simulink model "FP_sub_ML2017a"  (R2017a)
settings: Solver=FixedStepAuto  StartTime=0.0  StopTime=T  RelTol=1e-3  EnableMultiTasking=on
values from neighbouring files (symbols this model uses):
  Ts = 1    [Init.m]
libraries: My_FI_Operations x114, simulink x1
settings Model: FPTShortcutValueString='{{},{''BaselineRun'',1,1,1,''BaselineRun'','''',{},''M'',''D'',''''}}'  OrderedModelArguments=off  Creator=kavru  LastModifiedBy=kolbe
settings DataIOCC: ReturnWorkspaceOutputs=on
settings OptimizationCC: BlockReduction=off  ConditionallyExecuteInputs=off
settings DebuggingCC: SignalRangeChecking=warning  SingleTaskRateTransMsg=error
settings SFSimCC: SimUseLocalCustomCode=on
settings RTWCC: RTWUseLocalCustomCode=on

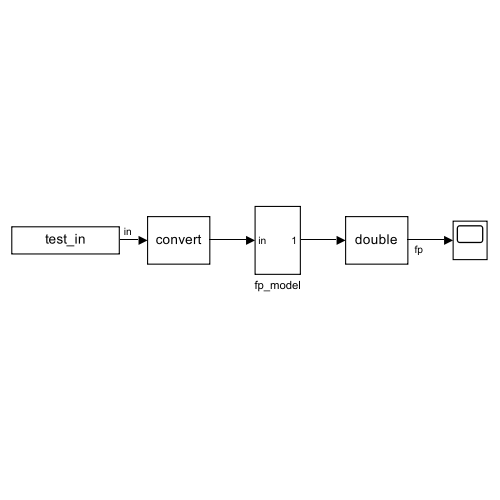
[thumbnail: Simulink's stored preview of the top-level diagram]
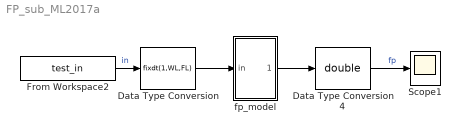
== system FP_sub_ML2017a ==
  Data Type Conversion : DataTypeConversion  OutDataTypeStr=fixdt(1,WL,FL)  RndMeth=Nearest  SaturateOnIntegerOverflow=on
  Data Type Conversion4 : DataTypeConversion  OutDataTypeStr=double  RndMeth=Nearest
  From Workspace2 : FromWorkspace  VariableName=test_in  OutDataTypeStr=double  SampleTime=Ts
  Scope1 : Scope
  fp_model : Subsystem
  wires:
  From Workspace2/1 -> Data Type Conversion/1  "in"
  fp_model/1(Out1) -> Data Type Conversion4/1
  Data Type Conversion/1 -> fp_model/1(in)
  Data Type Conversion4/1 -> Scope1/1  "fp"

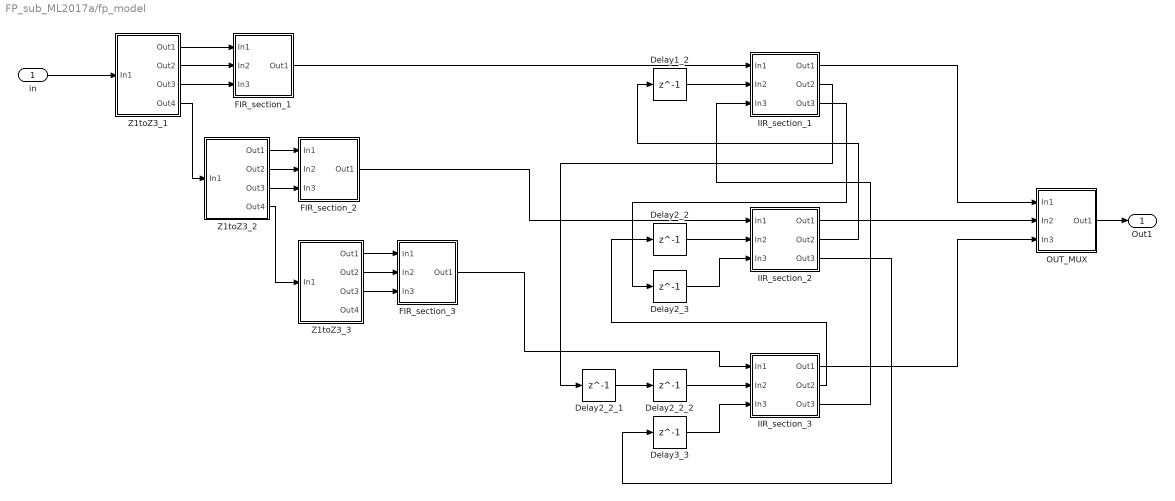
== system FP_sub_ML2017a/fp_model ==
  in : Inport
  Delay1_2 : Delay  DelayLength=1  SampleTime=3*Ts
  Delay2_2 : Delay  DelayLength=1  SampleTime=3*Ts
  Delay2_2_1 : Delay  DelayLength=1  SampleTime=3*Ts
  Delay2_2_2 : Delay  DelayLength=1  SampleTime=3*Ts
  Delay2_3 : Delay  DelayLength=1  SampleTime=3*Ts
  Delay3_3 : Delay  DelayLength=1  SampleTime=3*Ts
  FIR_section_1 : Subsystem
  FIR_section_2 : Subsystem
  FIR_section_3 : Subsystem
  IIR_section_1 : Subsystem
  IIR_section_2 : Subsystem
  IIR_section_3 : Subsystem
  OUT_MUX : Subsystem
  Z1toZ3_1 : Subsystem
  Z1toZ3_2 : Subsystem
  Z1toZ3_3 : Subsystem
  Out1 : Outport
  wires:
  in/1 -> Z1toZ3_1/1(In1)
  Z1toZ3_1/4(Out4) -> Z1toZ3_2/1(In1)
  Z1toZ3_2/4(Out4) -> Z1toZ3_3/1(In1)
  Z1toZ3_1/1(Out1) -> FIR_section_1/1(In1)
  Z1toZ3_1/2(Out2) -> FIR_section_1/2(In2)
  Z1toZ3_1/3(Out3) -> FIR_section_1/3(In3)
  Z1toZ3_2/1(Out1) -> FIR_section_2/1(In1)
  Z1toZ3_2/2(Out2) -> FIR_section_2/2(In2)
  Z1toZ3_2/3(Out3) -> FIR_section_2/3(In3)
  Z1toZ3_3/1(Out1) -> FIR_section_3/1(In1)
  Z1toZ3_3/2(Out2) -> FIR_section_3/2(In2)
  Z1toZ3_3/3(Out3) -> FIR_section_3/3(In3)
  OUT_MUX/1(Out1) -> Out1/1
  FIR_section_1/1(Out1) -> IIR_section_1/1(In1)
  Delay1_2/1 -> IIR_section_1/2(In2)
  IIR_section_1/1(Out1) -> OUT_MUX/1(In1)
  IIR_section_1/3(Out3) -> Delay2_3/1
  FIR_section_2/1(Out1) -> IIR_section_2/1(In1)
  Delay2_3/1 -> IIR_section_2/3(In3)
  Delay2_2/1 -> IIR_section_2/2(In2)
  IIR_section_2/1(Out1) -> OUT_MUX/2(In2)
  IIR_section_2/2(Out2) -> Delay1_2/1
  IIR_section_2/3(Out3) -> Delay3_3/1
  Delay2_2_2/1 -> IIR_section_3/2(In2)
  Delay3_3/1 -> IIR_section_3/3(In3)
  FIR_section_3/1(Out1) -> IIR_section_3/1(In1)
  IIR_section_3/3(Out3) -> IIR_section_1/3(In3)
  IIR_section_3/1(Out1) -> OUT_MUX/3(In3)
  IIR_section_3/2(Out2) -> Delay2_2/1
  Delay2_2_1/1 -> Delay2_2_2/1
  IIR_section_1/2(Out2) -> Delay2_2_1/1

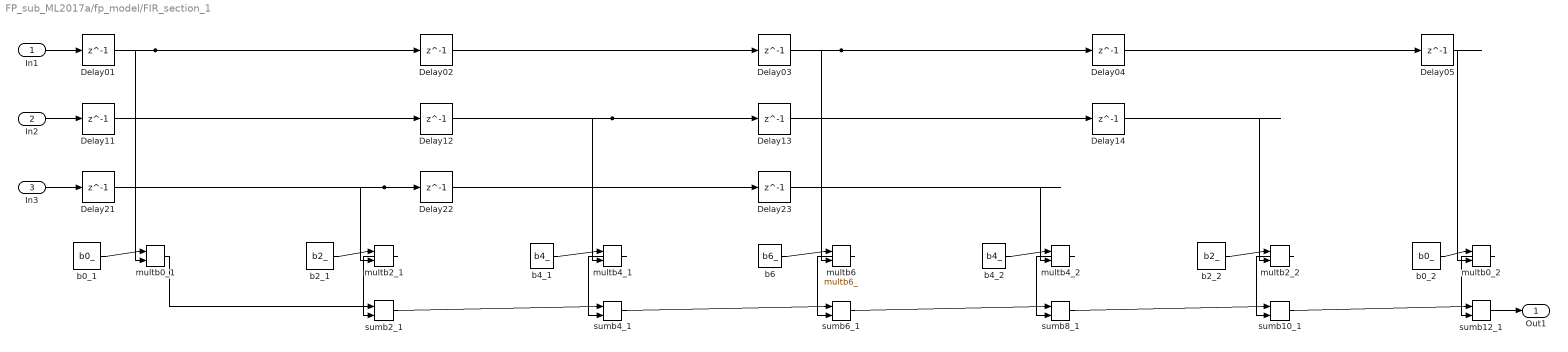
== system FP_sub_ML2017a/fp_model/FIR_section_1 ==
  In1 : Inport
  In2 : Inport  Port=2
  In3 : Inport  Port=3
  Delay01 : Delay  DelayLength=1  SampleTime=3*Ts
  Delay02 : Delay  DelayLength=1  SampleTime=3*Ts
  Delay03 : Delay  DelayLength=1  SampleTime=3*Ts
  Delay04 : Delay  DelayLength=1  SampleTime=3*Ts
  Delay05 : Delay  DelayLength=1  SampleTime=3*Ts
  Delay{11..14,21..23} (7 alike) : Delay  DelayLength=1  SampleTime=3*Ts
  b0_1 : My_FI_Operations/b0_  SystemSampleTime=-1  Latency=0  AutoFrameSizeCalculation=off
  b0_2 : My_FI_Operations/b0_  SystemSampleTime=-1  Latency=0  AutoFrameSizeCalculation=off
  b2_1 : My_FI_Operations/b2_  SystemSampleTime=-1  Latency=0  AutoFrameSizeCalculation=off
  b2_2 : My_FI_Operations/b2_  SystemSampleTime=-1  Latency=0  AutoFrameSizeCalculation=off
  b4_1 : My_FI_Operations/b4_  SystemSampleTime=-1  Latency=0  AutoFrameSizeCalculation=off
  b4_2 : My_FI_Operations/b4_  SystemSampleTime=-1  Latency=0  AutoFrameSizeCalculation=off
  b6 : My_FI_Operations/b6_  SystemSampleTime=-1  Latency=0  AutoFrameSizeCalculation=off
  multb0_1 : My_FI_Operations/multb0_  SystemSampleTime=-1  Latency=0  AutoFrameSizeCalculation=off
  multb0_2 : My_FI_Operations/multb0_  SystemSampleTime=-1  Latency=0  AutoFrameSizeCalculation=off
  multb2_1 : My_FI_Operations/multb2_  SystemSampleTime=-1  Latency=0  AutoFrameSizeCalculation=off
  multb2_2 : My_FI_Operations/multb2_  SystemSampleTime=-1  Latency=0  AutoFrameSizeCalculation=off
  multb4_1 : My_FI_Operations/multb4_  SystemSampleTime=-1  Latency=0  AutoFrameSizeCalculation=off
  multb4_2 : My_FI_Operations/multb4_  SystemSampleTime=-1  Latency=0  AutoFrameSizeCalculation=off
  multb6 : My_FI_Operations/multb6_  SystemSampleTime=-1  Latency=0  AutoFrameSizeCalculation=off
  sumb10_1 : My_FI_Operations/sumb10_  SystemSampleTime=-1  Latency=0  AutoFrameSizeCalculation=off
  sumb12_1 : My_FI_Operations/sumb12_  SystemSampleTime=-1  Latency=0  AutoFrameSizeCalculation=off
  sumb2_1 : My_FI_Operations/sumb2_  SystemSampleTime=-1  Latency=0  AutoFrameSizeCalculation=off
  sumb4_1 : My_FI_Operations/sumb4_  SystemSampleTime=-1  Latency=0  AutoFrameSizeCalculation=off
  sumb6_1 : My_FI_Operations/sumb6_  SystemSampleTime=-1  Latency=0  AutoFrameSizeCalculation=off
  sumb8_1 : My_FI_Operations/sumb8_  SystemSampleTime=-1  Latency=0  AutoFrameSizeCalculation=off
  Out1 : Outport
  wires:
  In3/1 -> Delay21/1
  Delay11/1 -> Delay12/1
  Delay01/1 -> multb0_1/2, Delay02/1
  Delay14/1 -> multb2_2/2
  Delay22/1 -> Delay23/1
  b2_2/1 -> multb2_2/1
  Delay23/1 -> multb4_2/2
  sumb6_1/1 -> sumb8_1/1
  multb2_1/1 -> sumb2_1/2
  Delay13/1 -> Delay14/1
  b0_2/1 -> multb0_2/1
  b0_1/1 -> multb0_1/1
  b4_2/1 -> multb4_2/1
  sumb8_1/1 -> sumb10_1/1
  multb0_2/1 -> sumb12_1/2
  Delay12/1 -> multb4_1/2, Delay13/1
  Delay02/1 -> Delay03/1
  Delay03/1 -> multb6/2, Delay04/1
  sumb4_1/1 -> sumb6_1/1
  multb4_1/1 -> sumb4_1/2
  b6/1 -> multb6/1
  Delay05/1 -> multb0_2/2
  b2_1/1 -> multb2_1/1
  b4_1/1 -> multb4_1/1
  sumb12_1/1 -> Out1/1
  multb6/1 -> sumb6_1/2
  multb0_1/1 -> sumb2_1/1
  multb4_2/1 -> sumb8_1/2
  Delay21/1 -> multb2_1/2, Delay22/1
  sumb2_1/1 -> sumb4_1/1
  In2/1 -> Delay11/1
  multb2_2/1 -> sumb10_1/2
  Delay04/1 -> Delay05/1
  sumb10_1/1 -> sumb12_1/1
  In1/1 -> Delay01/1

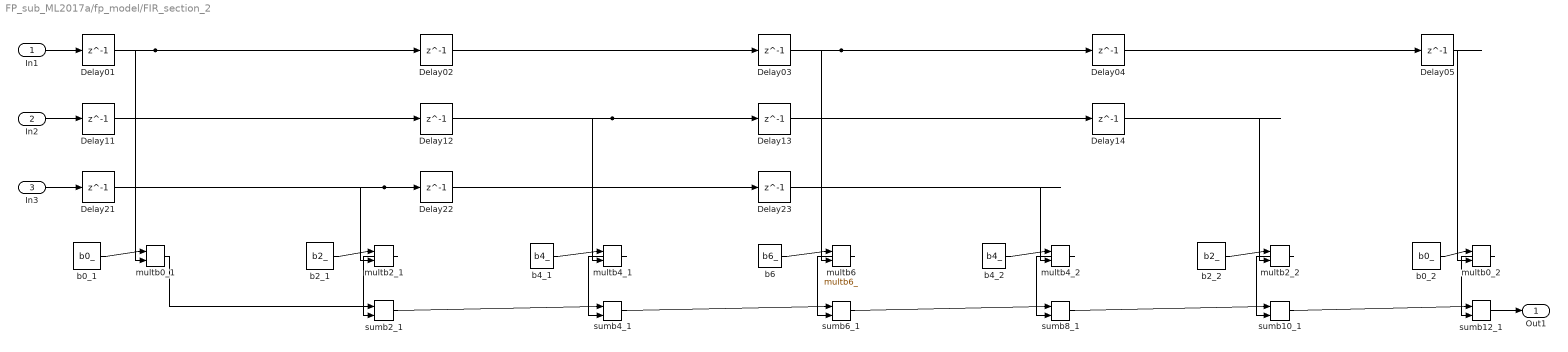
== system FP_sub_ML2017a/fp_model/FIR_section_2 ==
  In1 : Inport
  In2 : Inport  Port=2
  In3 : Inport  Port=3
  Delay01 : Delay  DelayLength=1  SampleTime=3*Ts
  Delay02 : Delay  DelayLength=1  SampleTime=3*Ts
  Delay03 : Delay  DelayLength=1  SampleTime=3*Ts
  Delay04 : Delay  DelayLength=1  SampleTime=3*Ts
  Delay05 : Delay  DelayLength=1  SampleTime=3*Ts
  Delay{11..14,21..23} (7 alike) : Delay  DelayLength=1  SampleTime=3*Ts
  b0_1 : My_FI_Operations/b0_  SystemSampleTime=-1  Latency=0  AutoFrameSizeCalculation=off
  b0_2 : My_FI_Operations/b0_  SystemSampleTime=-1  Latency=0  AutoFrameSizeCalculation=off
  b2_1 : My_FI_Operations/b2_  SystemSampleTime=-1  Latency=0  AutoFrameSizeCalculation=off
  b2_2 : My_FI_Operations/b2_  SystemSampleTime=-1  Latency=0  AutoFrameSizeCalculation=off
  b4_1 : My_FI_Operations/b4_  SystemSampleTime=-1  Latency=0  AutoFrameSizeCalculation=off
  b4_2 : My_FI_Operations/b4_  SystemSampleTime=-1  Latency=0  AutoFrameSizeCalculation=off
  b6 : My_FI_Operations/b6_  SystemSampleTime=-1  Latency=0  AutoFrameSizeCalculation=off
  multb0_1 : My_FI_Operations/multb0_  SystemSampleTime=-1  Latency=0  AutoFrameSizeCalculation=off
  multb0_2 : My_FI_Operations/multb0_  SystemSampleTime=-1  Latency=0  AutoFrameSizeCalculation=off
  multb2_1 : My_FI_Operations/multb2_  SystemSampleTime=-1  Latency=0  AutoFrameSizeCalculation=off
  multb2_2 : My_FI_Operations/multb2_  SystemSampleTime=-1  Latency=0  AutoFrameSizeCalculation=off
  multb4_1 : My_FI_Operations/multb4_  SystemSampleTime=-1  Latency=0  AutoFrameSizeCalculation=off
  multb4_2 : My_FI_Operations/multb4_  SystemSampleTime=-1  Latency=0  AutoFrameSizeCalculation=off
  multb6 : My_FI_Operations/multb6_  SystemSampleTime=-1  Latency=0  AutoFrameSizeCalculation=off
  sumb10_1 : My_FI_Operations/sumb10_  SystemSampleTime=-1  Latency=0  AutoFrameSizeCalculation=off
  sumb12_1 : My_FI_Operations/sumb12_  SystemSampleTime=-1  Latency=0  AutoFrameSizeCalculation=off
  sumb2_1 : My_FI_Operations/sumb2_  SystemSampleTime=-1  Latency=0  AutoFrameSizeCalculation=off
  sumb4_1 : My_FI_Operations/sumb4_  SystemSampleTime=-1  Latency=0  AutoFrameSizeCalculation=off
  sumb6_1 : My_FI_Operations/sumb6_  SystemSampleTime=-1  Latency=0  AutoFrameSizeCalculation=off
  sumb8_1 : My_FI_Operations/sumb8_  SystemSampleTime=-1  Latency=0  AutoFrameSizeCalculation=off
  Out1 : Outport
  wires:
  In3/1 -> Delay21/1
  Delay11/1 -> Delay12/1
  Delay01/1 -> multb0_1/2, Delay02/1
  Delay14/1 -> multb2_2/2
  Delay22/1 -> Delay23/1
  b2_2/1 -> multb2_2/1
  Delay23/1 -> multb4_2/2
  sumb6_1/1 -> sumb8_1/1
  multb2_1/1 -> sumb2_1/2
  Delay13/1 -> Delay14/1
  b0_2/1 -> multb0_2/1
  b0_1/1 -> multb0_1/1
  b4_2/1 -> multb4_2/1
  sumb8_1/1 -> sumb10_1/1
  multb0_2/1 -> sumb12_1/2
  Delay12/1 -> multb4_1/2, Delay13/1
  Delay02/1 -> Delay03/1
  Delay03/1 -> multb6/2, Delay04/1
  sumb4_1/1 -> sumb6_1/1
  multb4_1/1 -> sumb4_1/2
  b6/1 -> multb6/1
  Delay05/1 -> multb0_2/2
  b2_1/1 -> multb2_1/1
  b4_1/1 -> multb4_1/1
  sumb12_1/1 -> Out1/1
  multb6/1 -> sumb6_1/2
  multb0_1/1 -> sumb2_1/1
  multb4_2/1 -> sumb8_1/2
  Delay21/1 -> multb2_1/2, Delay22/1
  sumb2_1/1 -> sumb4_1/1
  In2/1 -> Delay11/1
  multb2_2/1 -> sumb10_1/2
  Delay04/1 -> Delay05/1
  sumb10_1/1 -> sumb12_1/1
  In1/1 -> Delay01/1

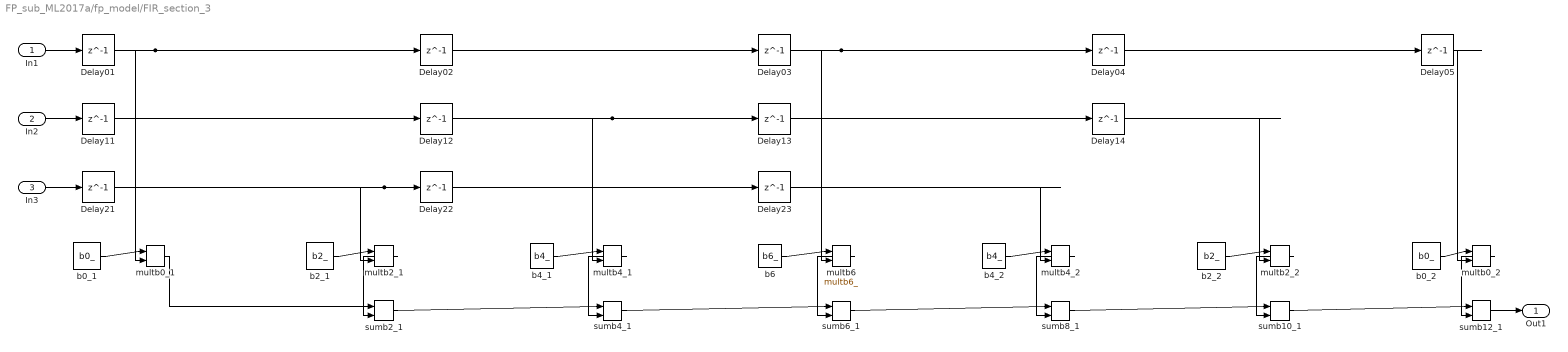
== system FP_sub_ML2017a/fp_model/FIR_section_3 ==
  In1 : Inport
  In2 : Inport  Port=2
  In3 : Inport  Port=3
  Delay01 : Delay  DelayLength=1  SampleTime=3*Ts
  Delay02 : Delay  DelayLength=1  SampleTime=3*Ts
  Delay03 : Delay  DelayLength=1  SampleTime=3*Ts
  Delay04 : Delay  DelayLength=1  SampleTime=3*Ts
  Delay05 : Delay  DelayLength=1  SampleTime=3*Ts
  Delay{11..14,21..23} (7 alike) : Delay  DelayLength=1  SampleTime=3*Ts
  b0_1 : My_FI_Operations/b0_  SystemSampleTime=-1  Latency=0  AutoFrameSizeCalculation=off
  b0_2 : My_FI_Operations/b0_  SystemSampleTime=-1  Latency=0  AutoFrameSizeCalculation=off
  b2_1 : My_FI_Operations/b2_  SystemSampleTime=-1  Latency=0  AutoFrameSizeCalculation=off
  b2_2 : My_FI_Operations/b2_  SystemSampleTime=-1  Latency=0  AutoFrameSizeCalculation=off
  b4_1 : My_FI_Operations/b4_  SystemSampleTime=-1  Latency=0  AutoFrameSizeCalculation=off
  b4_2 : My_FI_Operations/b4_  SystemSampleTime=-1  Latency=0  AutoFrameSizeCalculation=off
  b6 : My_FI_Operations/b6_  SystemSampleTime=-1  Latency=0  AutoFrameSizeCalculation=off
  multb0_1 : My_FI_Operations/multb0_  SystemSampleTime=-1  Latency=0  AutoFrameSizeCalculation=off
  multb0_2 : My_FI_Operations/multb0_  SystemSampleTime=-1  Latency=0  AutoFrameSizeCalculation=off
  multb2_1 : My_FI_Operations/multb2_  SystemSampleTime=-1  Latency=0  AutoFrameSizeCalculation=off
  multb2_2 : My_FI_Operations/multb2_  SystemSampleTime=-1  Latency=0  AutoFrameSizeCalculation=off
  multb4_1 : My_FI_Operations/multb4_  SystemSampleTime=-1  Latency=0  AutoFrameSizeCalculation=off
  multb4_2 : My_FI_Operations/multb4_  SystemSampleTime=-1  Latency=0  AutoFrameSizeCalculation=off
  multb6 : My_FI_Operations/multb6_  SystemSampleTime=-1  Latency=0  AutoFrameSizeCalculation=off
  sumb10_1 : My_FI_Operations/sumb10_  SystemSampleTime=-1  Latency=0  AutoFrameSizeCalculation=off
  sumb12_1 : My_FI_Operations/sumb12_  SystemSampleTime=-1  Latency=0  AutoFrameSizeCalculation=off
  sumb2_1 : My_FI_Operations/sumb2_  SystemSampleTime=-1  Latency=0  AutoFrameSizeCalculation=off
  sumb4_1 : My_FI_Operations/sumb4_  SystemSampleTime=-1  Latency=0  AutoFrameSizeCalculation=off
  sumb6_1 : My_FI_Operations/sumb6_  SystemSampleTime=-1  Latency=0  AutoFrameSizeCalculation=off
  sumb8_1 : My_FI_Operations/sumb8_  SystemSampleTime=-1  Latency=0  AutoFrameSizeCalculation=off
  Out1 : Outport
  wires:
  In3/1 -> Delay21/1
  Delay11/1 -> Delay12/1
  Delay01/1 -> multb0_1/2, Delay02/1
  Delay14/1 -> multb2_2/2
  Delay22/1 -> Delay23/1
  b2_2/1 -> multb2_2/1
  Delay23/1 -> multb4_2/2
  sumb6_1/1 -> sumb8_1/1
  multb2_1/1 -> sumb2_1/2
  Delay13/1 -> Delay14/1
  b0_2/1 -> multb0_2/1
  b0_1/1 -> multb0_1/1
  b4_2/1 -> multb4_2/1
  sumb8_1/1 -> sumb10_1/1
  multb0_2/1 -> sumb12_1/2
  Delay12/1 -> multb4_1/2, Delay13/1
  Delay02/1 -> Delay03/1
  Delay03/1 -> multb6/2, Delay04/1
  sumb4_1/1 -> sumb6_1/1
  multb4_1/1 -> sumb4_1/2
  b6/1 -> multb6/1
  Delay05/1 -> multb0_2/2
  b2_1/1 -> multb2_1/1
  b4_1/1 -> multb4_1/1
  sumb12_1/1 -> Out1/1
  multb6/1 -> sumb6_1/2
  multb0_1/1 -> sumb2_1/1
  multb4_2/1 -> sumb8_1/2
  Delay21/1 -> multb2_1/2, Delay22/1
  sumb2_1/1 -> sumb4_1/1
  In2/1 -> Delay11/1
  multb2_2/1 -> sumb10_1/2
  Delay04/1 -> Delay05/1
  sumb10_1/1 -> sumb12_1/1
  In1/1 -> Delay01/1

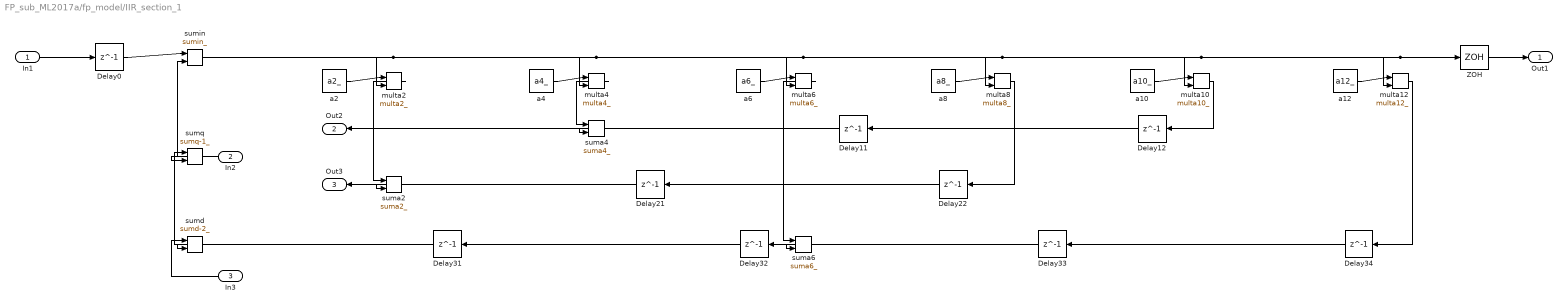
== system FP_sub_ML2017a/fp_model/IIR_section_1 ==
  In1 : Inport
  In2 : Inport  Port=2
  In3 : Inport  Port=3
  Delay{0,11..12,21..22,31..34} (9 alike) : Delay  DelayLength=1  SampleTime=3*Ts
  ZOH : ZeroOrderHold  SampleTime=3*Ts
  a10 : My_FI_Operations/a10_  SystemSampleTime=-1  Latency=0  AutoFrameSizeCalculation=off
  a12 : My_FI_Operations/a12_  SystemSampleTime=-1  Latency=0  AutoFrameSizeCalculation=off
  a2 : My_FI_Operations/a2_  SystemSampleTime=-1  Latency=0  AutoFrameSizeCalculation=off
  a4 : My_FI_Operations/a4_  SystemSampleTime=-1  Latency=0  AutoFrameSizeCalculation=off
  a6 : My_FI_Operations/a6_  SystemSampleTime=-1  Latency=0  AutoFrameSizeCalculation=off
  a8 : My_FI_Operations/a8_  SystemSampleTime=-1  Latency=0  AutoFrameSizeCalculation=off
  multa10 : My_FI_Operations/multa10_  SystemSampleTime=-1  Latency=0  AutoFrameSizeCalculation=off
  multa12 : My_FI_Operations/multa12_  SystemSampleTime=-1  Latency=0  AutoFrameSizeCalculation=off
  multa2 : My_FI_Operations/multa2_  SystemSampleTime=-1  Latency=0  AutoFrameSizeCalculation=off
  multa4 : My_FI_Operations/multa4_  SystemSampleTime=-1  Latency=0  AutoFrameSizeCalculation=off
  multa6 : My_FI_Operations/multa6_  SystemSampleTime=-1  Latency=0  AutoFrameSizeCalculation=off
  multa8 : My_FI_Operations/multa8_  SystemSampleTime=-1  Latency=0  AutoFrameSizeCalculation=off
  suma2 : My_FI_Operations/suma2_  SystemSampleTime=-1  Latency=0  AutoFrameSizeCalculation=off
  suma4 : My_FI_Operations/suma4_  SystemSampleTime=-1  Latency=0  AutoFrameSizeCalculation=off
  suma6 : My_FI_Operations/suma6_  SystemSampleTime=-1  Latency=0  AutoFrameSizeCalculation=off
  sumd : My_FI_Operations/sumd-2_  SystemSampleTime=-1  Latency=0  AutoFrameSizeCalculation=off
  sumin : My_FI_Operations/sumin_  SystemSampleTime=-1  Latency=0  AutoFrameSizeCalculation=off
  sumq : My_FI_Operations/sumq-1_  SystemSampleTime=-1  Latency=0  AutoFrameSizeCalculation=off
  Out1 : Outport
  Out2 : Outport  Port=2
  Out3 : Outport  Port=3
  wires:
  Delay0/1 -> sumin/1
  a12/1 -> multa12/1
  Delay22/1 -> Delay21/1
  Delay31/1 -> sumd/2
  sumin/1 -> multa2/2, multa4/2, multa6/2, multa8/2, multa10/2, multa12/2, ZOH/1
  Delay33/1 -> suma6/2
  Delay32/1 -> Delay31/1
  Delay21/1 -> suma2/2
  sumd/1 -> sumq/1
  a2/1 -> multa2/1
  multa4/1 -> suma4/1
  Delay12/1 -> Delay11/1
  ZOH/1 -> Out1/1
  multa6/1 -> suma6/1
  a10/1 -> multa10/1
  a4/1 -> multa4/1
  multa12/1 -> Delay34/1
  multa2/1 -> suma2/1
  Delay34/1 -> Delay33/1
  a8/1 -> multa8/1
  suma6/1 -> Delay32/1
  Delay11/1 -> suma4/2
  multa10/1 -> Delay12/1
  multa8/1 -> Delay22/1
  sumq/1 -> sumin/2
  a6/1 -> multa6/1
  In2/1 -> sumq/2
  In1/1 -> Delay0/1
  In3/1 -> sumd/1
  suma2/1 -> Out3/1
  suma4/1 -> Out2/1

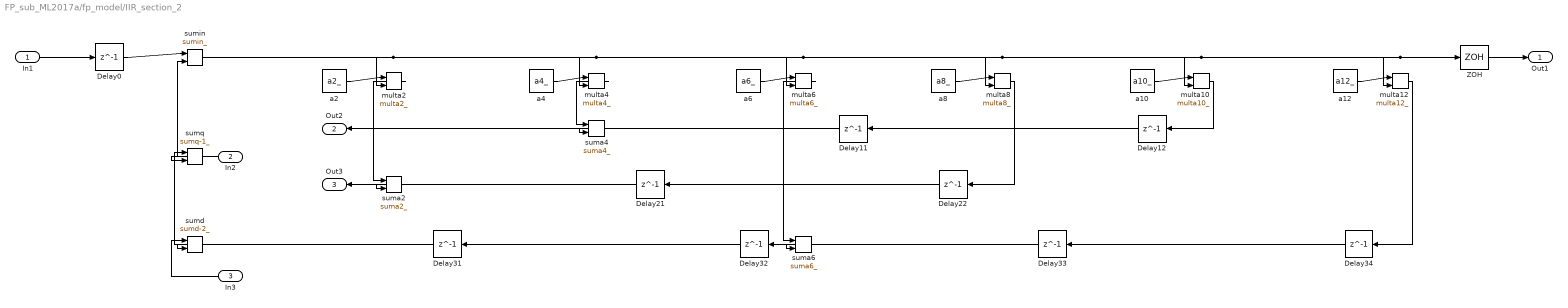
== system FP_sub_ML2017a/fp_model/IIR_section_2 ==
  In1 : Inport
  In2 : Inport  Port=2
  In3 : Inport  Port=3
  Delay{0,11..12,21..22,31..34} (9 alike) : Delay  DelayLength=1  SampleTime=3*Ts
  ZOH : ZeroOrderHold  SampleTime=3*Ts
  a10 : My_FI_Operations/a10_  SystemSampleTime=-1  Latency=0  AutoFrameSizeCalculation=off
  a12 : My_FI_Operations/a12_  SystemSampleTime=-1  Latency=0  AutoFrameSizeCalculation=off
  a2 : My_FI_Operations/a2_  SystemSampleTime=-1  Latency=0  AutoFrameSizeCalculation=off
  a4 : My_FI_Operations/a4_  SystemSampleTime=-1  Latency=0  AutoFrameSizeCalculation=off
  a6 : My_FI_Operations/a6_  SystemSampleTime=-1  Latency=0  AutoFrameSizeCalculation=off
  a8 : My_FI_Operations/a8_  SystemSampleTime=-1  Latency=0  AutoFrameSizeCalculation=off
  multa10 : My_FI_Operations/multa10_  SystemSampleTime=-1  Latency=0  AutoFrameSizeCalculation=off
  multa12 : My_FI_Operations/multa12_  SystemSampleTime=-1  Latency=0  AutoFrameSizeCalculation=off
  multa2 : My_FI_Operations/multa2_  SystemSampleTime=-1  Latency=0  AutoFrameSizeCalculation=off
  multa4 : My_FI_Operations/multa4_  SystemSampleTime=-1  Latency=0  AutoFrameSizeCalculation=off
  multa6 : My_FI_Operations/multa6_  SystemSampleTime=-1  Latency=0  AutoFrameSizeCalculation=off
  multa8 : My_FI_Operations/multa8_  SystemSampleTime=-1  Latency=0  AutoFrameSizeCalculation=off
  suma2 : My_FI_Operations/suma2_  SystemSampleTime=-1  Latency=0  AutoFrameSizeCalculation=off
  suma4 : My_FI_Operations/suma4_  SystemSampleTime=-1  Latency=0  AutoFrameSizeCalculation=off
  suma6 : My_FI_Operations/suma6_  SystemSampleTime=-1  Latency=0  AutoFrameSizeCalculation=off
  sumd : My_FI_Operations/sumd-2_  SystemSampleTime=-1  Latency=0  AutoFrameSizeCalculation=off
  sumin : My_FI_Operations/sumin_  SystemSampleTime=-1  Latency=0  AutoFrameSizeCalculation=off
  sumq : My_FI_Operations/sumq-1_  SystemSampleTime=-1  Latency=0  AutoFrameSizeCalculation=off
  Out1 : Outport
  Out2 : Outport  Port=2
  Out3 : Outport  Port=3
  wires:
  Delay0/1 -> sumin/1
  a12/1 -> multa12/1
  Delay22/1 -> Delay21/1
  Delay31/1 -> sumd/2
  sumin/1 -> multa2/2, multa4/2, multa6/2, multa8/2, multa10/2, multa12/2, ZOH/1
  Delay33/1 -> suma6/2
  Delay32/1 -> Delay31/1
  Delay21/1 -> suma2/2
  sumd/1 -> sumq/1
  a2/1 -> multa2/1
  multa4/1 -> suma4/1
  Delay12/1 -> Delay11/1
  ZOH/1 -> Out1/1
  multa6/1 -> suma6/1
  a10/1 -> multa10/1
  a4/1 -> multa4/1
  multa12/1 -> Delay34/1
  multa2/1 -> suma2/1
  Delay34/1 -> Delay33/1
  a8/1 -> multa8/1
  suma6/1 -> Delay32/1
  Delay11/1 -> suma4/2
  multa10/1 -> Delay12/1
  multa8/1 -> Delay22/1
  sumq/1 -> sumin/2
  a6/1 -> multa6/1
  In2/1 -> sumq/2
  In1/1 -> Delay0/1
  In3/1 -> sumd/1
  suma2/1 -> Out3/1
  suma4/1 -> Out2/1

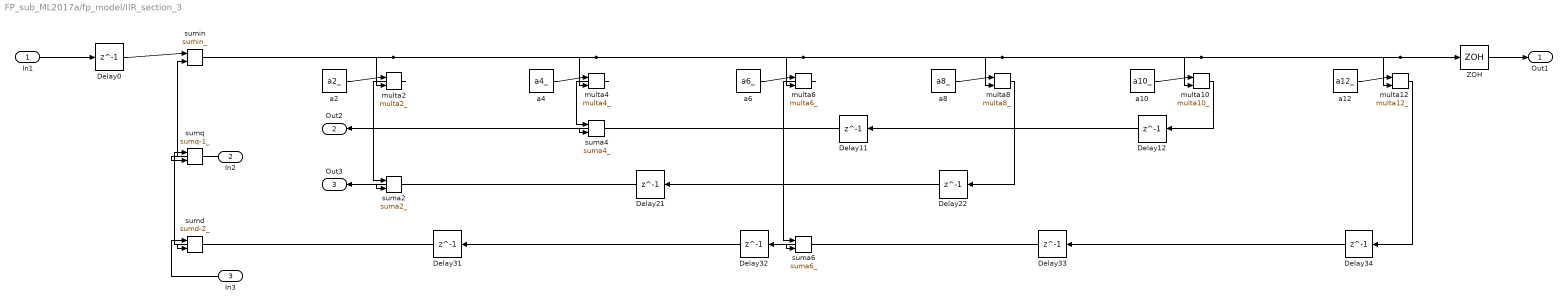
== system FP_sub_ML2017a/fp_model/IIR_section_3 ==
  In1 : Inport
  In2 : Inport  Port=2
  In3 : Inport  Port=3
  Delay{0,11..12,21..22,31..34} (9 alike) : Delay  DelayLength=1  SampleTime=3*Ts
  ZOH : ZeroOrderHold  SampleTime=3*Ts
  a10 : My_FI_Operations/a10_  SystemSampleTime=-1  Latency=0  AutoFrameSizeCalculation=off
  a12 : My_FI_Operations/a12_  SystemSampleTime=-1  Latency=0  AutoFrameSizeCalculation=off
  a2 : My_FI_Operations/a2_  SystemSampleTime=-1  Latency=0  AutoFrameSizeCalculation=off
  a4 : My_FI_Operations/a4_  SystemSampleTime=-1  Latency=0  AutoFrameSizeCalculation=off
  a6 : My_FI_Operations/a6_  SystemSampleTime=-1  Latency=0  AutoFrameSizeCalculation=off
  a8 : My_FI_Operations/a8_  SystemSampleTime=-1  Latency=0  AutoFrameSizeCalculation=off
  multa10 : My_FI_Operations/multa10_  SystemSampleTime=-1  Latency=0  AutoFrameSizeCalculation=off
  multa12 : My_FI_Operations/multa12_  SystemSampleTime=-1  Latency=0  AutoFrameSizeCalculation=off
  multa2 : My_FI_Operations/multa2_  SystemSampleTime=-1  Latency=0  AutoFrameSizeCalculation=off
  multa4 : My_FI_Operations/multa4_  SystemSampleTime=-1  Latency=0  AutoFrameSizeCalculation=off
  multa6 : My_FI_Operations/multa6_  SystemSampleTime=-1  Latency=0  AutoFrameSizeCalculation=off
  multa8 : My_FI_Operations/multa8_  SystemSampleTime=-1  Latency=0  AutoFrameSizeCalculation=off
  suma2 : My_FI_Operations/suma2_  SystemSampleTime=-1  Latency=0  AutoFrameSizeCalculation=off
  suma4 : My_FI_Operations/suma4_  SystemSampleTime=-1  Latency=0  AutoFrameSizeCalculation=off
  suma6 : My_FI_Operations/suma6_  SystemSampleTime=-1  Latency=0  AutoFrameSizeCalculation=off
  sumd : My_FI_Operations/sumd-2_  SystemSampleTime=-1  Latency=0  AutoFrameSizeCalculation=off
  sumin : My_FI_Operations/sumin_  SystemSampleTime=-1  Latency=0  AutoFrameSizeCalculation=off
  sumq : My_FI_Operations/sumq-1_  SystemSampleTime=-1  Latency=0  AutoFrameSizeCalculation=off
  Out1 : Outport
  Out2 : Outport  Port=2
  Out3 : Outport  Port=3
  wires:
  Delay0/1 -> sumin/1
  a12/1 -> multa12/1
  Delay22/1 -> Delay21/1
  Delay31/1 -> sumd/2
  sumin/1 -> multa2/2, multa4/2, multa6/2, multa8/2, multa10/2, multa12/2, ZOH/1
  Delay33/1 -> suma6/2
  Delay32/1 -> Delay31/1
  Delay21/1 -> suma2/2
  sumd/1 -> sumq/1
  a2/1 -> multa2/1
  multa4/1 -> suma4/1
  Delay12/1 -> Delay11/1
  ZOH/1 -> Out1/1
  multa6/1 -> suma6/1
  a10/1 -> multa10/1
  a4/1 -> multa4/1
  multa12/1 -> Delay34/1
  multa2/1 -> suma2/1
  Delay34/1 -> Delay33/1
  a8/1 -> multa8/1
  suma6/1 -> Delay32/1
  Delay11/1 -> suma4/2
  multa10/1 -> Delay12/1
  multa8/1 -> Delay22/1
  sumq/1 -> sumin/2
  a6/1 -> multa6/1
  In2/1 -> sumq/2
  In1/1 -> Delay0/1
  In3/1 -> sumd/1
  suma2/1 -> Out3/1
  suma4/1 -> Out2/1

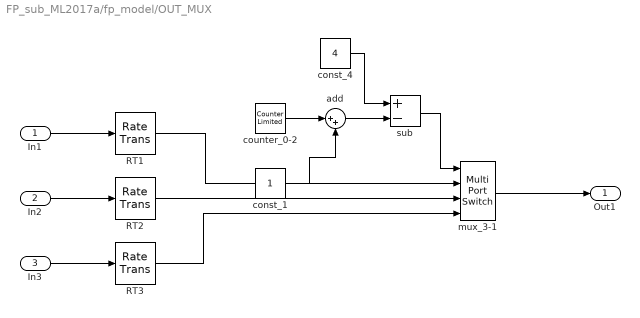
== system FP_sub_ML2017a/fp_model/OUT_MUX ==
  In1 : Inport
  In2 : Inport  Port=2
  In3 : Inport  Port=3
  RT1 : RateTransition  OutPortSampleTime=Ts
  RT2 : RateTransition  OutPortSampleTime=Ts
  RT3 : RateTransition  OutPortSampleTime=Ts
  add : Sum  Inputs=|++  OutDataTypeStr=fixdt(0,2,0)
  const_1 : Constant  OutDataTypeStr=fixdt(0,1,0)
  const_4 : Constant  Value=4  OutDataTypeStr=fixdt(0,3,0)
  counter_0-2 : simulink/Sources/Counter Limited  uplimit=2  tsamp=Ts
  mux_3-1 : MultiPortSwitch  OutDataTypeStr=fixdt(1,WL,FLout)  RndMeth=Nearest
  sub : Sum  Inputs=+-  OutDataTypeStr=fixdt(0,2,0)
  Out1 : Outport
  wires:
  RT3/1 -> mux_3-1/4
  const_1/1 -> add/2
  sub/1 -> mux_3-1/1
  counter_0-2/1 -> add/1
  add/1 -> sub/2
  const_4/1 -> sub/1
  RT1/1 -> mux_3-1/2
  RT2/1 -> mux_3-1/3
  In2/1 -> RT2/1
  In1/1 -> RT1/1
  mux_3-1/1 -> Out1/1
  In3/1 -> RT3/1

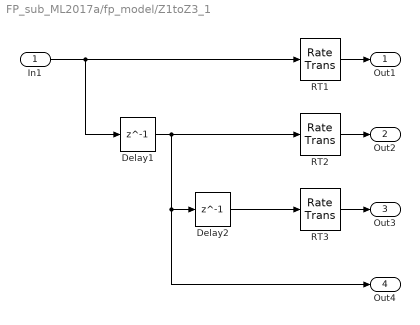
== system FP_sub_ML2017a/fp_model/Z1toZ3_1 ==
  In1 : Inport
  Delay1 : Delay  DelayLength=1  SampleTime=Ts
  Delay2 : Delay  DelayLength=1  SampleTime=Ts
  RT1 : RateTransition  OutPortSampleTime=3*Ts
  RT2 : RateTransition  OutPortSampleTime=3*Ts
  RT3 : RateTransition  OutPortSampleTime=3*Ts
  Out1 : Outport
  Out2 : Outport  Port=2
  Out3 : Outport  Port=3
  Out4 : Outport  Port=4
  wires:
  Delay1/1 -> RT2/1, Out4/1, Delay2/1
  Delay2/1 -> RT3/1
  In1/1 -> Delay1/1, RT1/1
  RT1/1 -> Out1/1
  RT2/1 -> Out2/1
  RT3/1 -> Out3/1

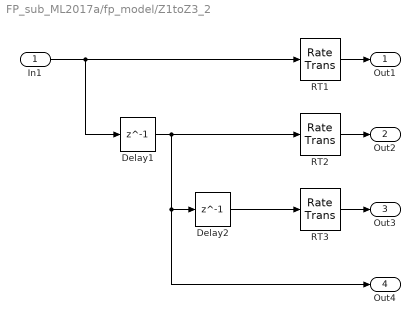
== system FP_sub_ML2017a/fp_model/Z1toZ3_2 ==
  In1 : Inport
  Delay1 : Delay  DelayLength=1  SampleTime=Ts
  Delay2 : Delay  DelayLength=1  SampleTime=Ts
  RT1 : RateTransition  OutPortSampleTime=3*Ts
  RT2 : RateTransition  OutPortSampleTime=3*Ts
  RT3 : RateTransition  OutPortSampleTime=3*Ts
  Out1 : Outport
  Out2 : Outport  Port=2
  Out3 : Outport  Port=3
  Out4 : Outport  Port=4
  wires:
  Delay1/1 -> RT2/1, Out4/1, Delay2/1
  Delay2/1 -> RT3/1
  In1/1 -> Delay1/1, RT1/1
  RT1/1 -> Out1/1
  RT2/1 -> Out2/1
  RT3/1 -> Out3/1

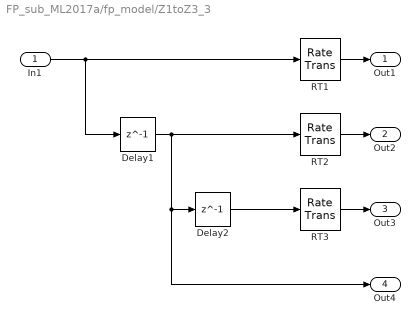
== system FP_sub_ML2017a/fp_model/Z1toZ3_3 ==
  In1 : Inport
  Delay1 : Delay  DelayLength=1  SampleTime=Ts
  Delay2 : Delay  DelayLength=1  SampleTime=Ts
  RT1 : RateTransition  OutPortSampleTime=3*Ts
  RT2 : RateTransition  OutPortSampleTime=3*Ts
  RT3 : RateTransition  OutPortSampleTime=3*Ts
  Out1 : Outport
  Out2 : Outport  Port=2
  Out3 : Outport  Port=3
  Out4 : Outport  Port=4
  wires:
  Delay1/1 -> RT2/1, Out4/1, Delay2/1
  Delay2/1 -> RT3/1
  In1/1 -> Delay1/1, RT1/1
  RT1/1 -> Out1/1
  RT2/1 -> Out2/1
  RT3/1 -> Out3/1
